simulink library "ann"  (Simulink 3.00)
undefined symbols (not defined in the file): V0, W0
libraries: simulink3 x3, neural x1
(part 1 of 2)
settings Model: LastModifiedBy=campa

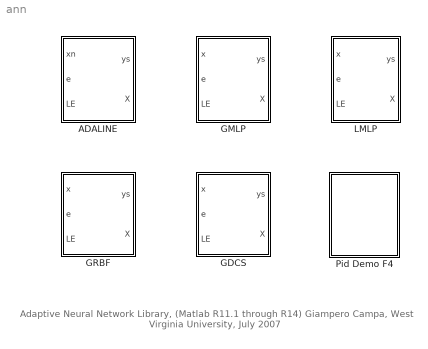
== system ann ==
  note: Adaptive Neural Network Library, (Matlab R11.1 through R14)
      | Giampero Campa, West Virginia University, July 2007
  ADALINE : Subsystem  mask(Adaline NN){dim=[4 1], eta=0.1, gam=1e-6, L=Inf, W=0, T=0.05}
      mask prompts: dim "[ni no]"; eta "Learning Rate"; gam "Stabilizing Factor"; L "Weight Limiter"; W "Initial Condition"; T "Sample Time"
      mask help: Self Adaptive Discrete Time MIMO Linear Neural Network
      mask init:
      | ni=dim(1);no=dim(2);
      mask Help:
      | <p>
      |   This Neural Network is used to adaptively approximate
      |   an affine vector field y=W*x+k, with the input vector
      |   x being a function of time.
      | </p>
      | <p>
      |   The first input is x. <br>
      |   The second input is the error signal (i.e. e=y-ys). <br>
      |   The third input is the learning enable:
      |        with LE=1 the learning is enabled,
      |        with LE=0 the learning is disabled.
      | </p>
      | <p>
      |   The first output is the learned function ys(x). <br>
      |   The second output is the states matrix reshaped columnwise. <br>
      | </p>
      | <p>
      |   The first parameter in the mask is a vector containing Ni and No,
      |   namely the dimensions (number of elements) of x and y.
      | </p>
      | <p>
      |   The second parameter in the mask is the learning rate.
      | </p>
      | <p>
      |   The third parameter in the mask is the stabilizing factor.
      | </p>
      | <p>
      |   The fourth parameter in the mask is a limiter for each element of the weight matrix.
      | </p>
      | <p>
      |   The initial condition could be either a vector of No*(Ni+1)
      |   parameters or a scalar. In the latter case, the scalar
      |   is repeated No*(Ni+1) times to form the initial condition vector.
      | </p>
      | <p>
      |   OUTPUT EQUATION: <br>
      |   At any given time t, if x(t) is the input vector,
      |   then the h-th output of the neural network is : <br>
      |   ys(h,t)=0.1*Wo(h,t)+Ws(h,t)*x(t) <br>
      |   where Wo(h,t) and Ws(h,t) are respectively the first element
      |   and the rest of the h-th row of the state matrix W(t). <br>
      | <br>
      |   STATE EQUATION (Learning Algorithm): <br>
      |   The state matrix W(t) is updated according to the gradient rule:
      |   W(t+T)=W(t)+eta*(dys/dW)*e(t)-eta*gamma*W(t) <br>
      |   where eta is the learning rate, dys/dW is a jacobian matrix,
      |   gamma is the stabilizing factor (sigma modification),
      |   e(t)=y(t)-ys(t) is the error vector at time t, and T is the sampling time.
      | </p>
      | <p>
      |   The final mask parameter is the sampling time of the block, T.
      | </p>
      | <p>
      |   This block is implemented in Simulink,
      |   to use it you should have the smxl library in your path.
      |   For further reference see some papers on the ADALINE NN.<br>
      | </p>
      | <p>
      |   Giampiero Campa, June 20 2003
      | </p>
  GDCS : Subsystem  mask(GDCS NN){Dim=[4 1], norlat=[50     0.2        0.01    600       0.99    0.005], eta=[0.03  0.003  0.1  0.001   0 ], lim=[1 1 1]*1e6, lga=on, S=zeros(1*(50*(50+4+5)+2),1), T=0.05}
      mask prompts: Dim "[Ni No]"; norlat "[Nmax Overlap RsThr Lambda Alpha Theta]"; eta "[Epsb Epsn etaW etaS etaC]"; lim "[limW limS limC]"; lga "Piecewise Conical Activation Function (otherwise Gaussian)"; S "Initial Condition, size = (Nmax*(Nmax+Ni+5)+2)*No"; T "Sample Time"
      mask help: Self Adaptive Discrete Time Generalized DCS Neural Network
      mask init:
      | if prod(size(Dim))==1,Dim=[Dim 1]; end
      mask Help:
      | <p>
      |   This Neural Network is used to adaptively approximate
      |   a vector field y=f(x), where x(t) is a vector of size Ni,
      |   and y(t) is a vector of size No.
      | </p>
      | <p>
      |   The first input is x (normally but not necessarily
      |   scaled between -1 and 1).<br>
      |   The second input is the error signal (i.e. e=y-ys).<br>
      |   The third input is the learning enable:
      |        with LE=1 the learning is enabled,
      |        with LE=0 the learning is disabled.
      | </p>
      | <p>
      |   The first output is the learned function ys(x). <br>
      |   The second output is the states matrix reshaped columnwise.
      |   Note that the network has in total No*(Nmax*(Nmax+Ni+5)+2) states,
      |   where Nmax is the maximum number of neurons per output.
      | </p>
      | <p>
      |   The first parameter in the mask is a vector containing Ni and No,
      |   namely the dimensions (number of elements) of x and y.
      | </p>
      | <p>
      |   The second parameter is a vector containing:<br>
      |   1) Nmax : the maximum number of active neurons for a single output.
      |       The total maximum number of active neurons in the whole network
      |       is this value multplied by the number of outputs, that is Nmax*No. <br>
      |   2) Overlapping Factor (when a new neuron is activated, the sigma (width) of
      |       this new neuron, is the sum of the distances from the two nearest
      |       neurons multiplied by the overlapping factor). <br>
      |   3) Resource Threshold, a new neuron is added only if the
      |       resource is greater than than this threshold. <br>
      |   4) Lambda, is the number of steps between insertion,
      |       a new neuron is activated only if the number of steps
      |       from the last activation is greater than lambda. <br>
      |   5) Alpha, is the connection weight decay constant
      |       for the neighborhood of the best matching unit.<br>
      |   6) Theta is the connection deletion threshold, that is when
      |       the weight falls below this threshold, it is set to 0,
      |       so the neuron is deactivated.
      | </p>
      | <p>
      |   The third parameters is 5 elements vector containing : <br>
      |   1) The two Kohonen update coefficients for the best
      |   matching unit and its neighborhood <br>
      |   2) the three learning rates for all the neurons states:
      |   weights, sigmas, and centers.
      | </p>
      | <p>
      |   The fifth parameter contains 3 limits for each element of the weight,
      |    sigma and center matrices. Basically, a limiting mechanism is implemented
      |    within the code so that the norms of each element of the weight, sigma
      |    and center vectors are confined within the upper bound entered as    parameter.
      | </p>
      | <p>
      |   The fifth parameter decides wether the activation function is
      |    piecewise conical or gaussian
      | </p>
      | <p>
      |   The initial condition must be a vector of size
      |   No*(Nmax*(Nmax+Ni+5)+2). If its norm is zero, then an
      |   appropriate initial condition (two neurons near zero) is chosen.
      | </p>
      | <p>
      |   STATE VECTOR MEANING: <br>
      |   Each output h is related to a contiguous vector of Nmax*(Nmax+Ni+5)+2
      |   states that are organized as follows: <br>
      |   ofY + 1 counter :  counts sampling times since last neuron activation. <br>
      |   ofY + 1 + [1..Nmax*Nmax] : interlayer connection matrix. <br>
      |   ofY + 1 + Nmax*Nmax + [1..Nmax*Ni] : neurons centers <br>
      |   ofY + 1 + Nmax*(Nmax+Ni) + [1..Nmax]: neurons weigths <br>
      |   ofY + 1 + Nmax*(Nmax+Ni+1) + [1..Nmax] : neurons sigmas (widths) <br>
      |   ofY + 1 + Nmax*(Nmax+Ni+2) + [1..Nmax] : neurons cumulative resource <br>
      |   ofY + 1 + Nmax*(Nmax+Ni+3) + [1..Nmax] : neurons resource<br>
      |   ofY + 1 + Nmax*(Nmax+Ni+4) + [1..Nmax] : number of times that each neuron has been bmu <br>
      |   ofY + 1 + Nmax*(Nmax+Ni+5) + 1 : number of active neurons <br>
      |   where ofY=(h-1)*(Nmax*(Nmax+Ni+5)+2) is the offset related to the h-th output.<br>
      |   It is important to note that the states related to a certain output
      |   are independent from the states related to a different output.
      |   Also note that the states related to the sigmas are only used for gaussian activation functions.
      | </p>
      | <p>
      |   BRIEF EXPLANATION OF THE ALGORITHM: <br>
      |   This Neural Network is essentially an RBF Neural Network with an
      |   additional lateral connection structure between the neural units
      |   of the hidden layer. This structure is used in an attempt to mirror
      |   the topology of the input manifold. <br>
      |   As in the RAN, the learning algorithm, in order to decrease the error,
      |   changes weights, positions and widths of the basis functions.
      |   The estimation error e(k) is accumulated locally to each neuron and
      |   used to determine where (and if) to activate a new neuron. <br>
      |   DSC stands for Dynamic Cell Structure.<br>
      | <br>
      |   OUTPUT EQUATION: <br>
      | At any given time t, if x(t) is the input vector, we indicate with bmu the nearest unit (among those related to the h-th output) to the current position of the input, and with sec is the nearest unit after the bmu. The neighborhood of the bmu is defined as the set of all the units that are connected to the bmu
      | by the interlayer connection matrix CN, that is all the units i such that CN(h,t,bmu,i) > 0.
      | Being W(h,t,bmu) and W(h,t,sec) the weights associated with the bmu and the sec units, and dist(bmu,x)  and dist(sec,x) their distances from the current input point x(t), if the PIECEWISE CONICAL activation functions are used, then the h-th output of the neural network is :
      | ys(h,t)=W(h,t,bmu) if dist(sec,x)>dist(sec,bmu)
      | ys(h,t)=W(h,t,bmu)+b*(W(h,t,sec)-W(h,t,bmu)) otherwise
      | where b=dist(bmu,x)/(dist(bmu,x)+dist(sec,x))
      | <br>
      |   If the GAUSSIAN activation functions are used t, then the h-th output
      |   of the neural network is simply: <br>
      |   ys(h,t)=W(h,t)*g(x(t),S(h,t),C(h,t)) <br>
      |   where W(h,t) is the output weight matrix related to the h-th output,
      |   g is the vector of radial basis functions of the input x(t), and
      |   finally S(h,t) and C(h,t) are vectors of widths and centers
      |   (relative to the h-th output).<br>
      | <br>
      |   STATE EQUATION (Learning Algorithm): <br>
      |   Being e(h,t)=y(h,t)-ys(h,t) the h-th element of the error vector,
      |   at a time t, and x(t) the input vector at the same time, we indicate
      |   with bmu the nearest unit (among those related to the h-th output)
      |   to the current position of the input, and with sec is the nearest
      |   unit after the bmu. The neighborhood of the bmu is defined as the set of
      |   all the units that are connected to the bmu by the interlayer connection
      |   matrix CN, that is all the units i such that CN(h,t,bmu,i) > 0. <br>
      |   Firstly, the connection matrix updated, by setting to 1 the strength of
      |   the connection between bmu and sec, ( that is CN(h,t+1,bmu,sec)=1 and
      |   CN(h,t+1,sec,bmu)=1 ), and by multiplying by a value alpha < 1 the
      |   strength of all the other connections ( that is for every i,j <> bmu,sec
      |   CN(h,t+1,i,j)=CN(h,t,i,j)*alpha ). Also, all the connections whose
      |   strength is less than a threshold theta are deleted (i.e. their strength
      |   is set to 0). This kind of updating is also called "Hebbian Learning". <br>
      |   The next step in the network adaptation algorithm consist in moving the
      |   positions of the BMU and its neighborhood toward the current input x(t),
      |   following a so called "Kohonen" rule. Specifically, if C(h,t,i) is
      |   the position of the neuron i, related to the output h, at time t,
      |   then for each neuron i belonging to the neighborhood of the bmu
      |   we have C(h,t+1,i)=epsilon(i)*(x(t)-C(h,t,i)). <br>
      |   Each neuron i is associated with a value called resource, R(h,t,i) and
      |   at this point in the algorithm, the resource of the bmu is updated,
      |   specifically, the resource of the bmu is set to the error e(h,t)
      |   divided by the number of times that the unit has been selected as bmu. <br>
      |   If the mean value of the resource of the whole network is greater than
      |   a certain threshold RsThr, and if the last neuron activation was more than
      |   lambda steps ago, then a new neuron is activated. <br>
      |   The new neuron n is placed between the position of the unit with highest
      |   resource w and the position of the unit with highest resource within the
      |   neighborhood of w, excluding w itself, let us indicate it with v.
      |   In detail, C(h,t+1,n)=C(h,t,w)+b*(C(h,t,v)-C(h,t,w)), where
      |   b=R(h,t,w)/(R(h,t,w)+R(h,t,v)). <br>
      |   The interlayer connections from w to n and from n to v are set to 1,
      |   the original connection between w and v is set to 0. Both resource and
      |   weight of the new neuron are computed by interpolating the resource and
      |   weight of the two neurons w and v:  <br>
      |   R(h,t+1,n)=R(h,t,w)+b*(R(h,t,v)-R(h,t,w)) <br>
      |   W(h,t+1,n)=W(h,t,w)+b*(W(h,t,v)-W(h,t,w)) <br>
      |   The width of the basis function of n is set to
      |   S(h,t,n)=overlap*(C(h,t,v)-C(h,t,w)), where overlap is the so called
      |   overlapping factor. <br>
      |   Finally, as a last step of the adaptation algorithm, the vector X(t)
      |   containing all the neural network weights and widths,
      |   is updated according to the gradient rule: <br>
      |   X(t+T)=X(t)+eta*(dys/dX)*e(t) <br>
      |   where eta is the learning rate, dys/dX is a jacobian matrix,
      |   and T is the sampling time.
      | </p>
      | <p>
      |   The final mask parameter is the sampling time of the block, T.
      | </p>
      | <p>
      |   This block calls the mex file obtained by compiling the s-function
      |   dcsgl.c, therefore, to use the block, you should have the resulting
      |   mex file (on windows platform the file is dcsgl.dll) in the matlab path.<br>
      |   For further reference see some papers on DSC Networks.<br>
      | </p>
      | <p>
      |   Giampiero Campa, January 2007
      | </p>
  GMLP : Subsystem  mask(GMLP NN){dim=[4 10 1], eta=[0.003 0.003 0.003]/10, L=[inf inf inf], alp=0.01, ini=1, T=0.05}
      mask prompts: dim "[ni nh no]"; eta "[etaV etaW etaP]"; L "[Lv Lw Lp] (Weight Limiters)"; alp "Momentum (alpha)"; ini "Initial Conditions"; T "Sample Time"
      mask help: Self Adaptive Discrete Time Generalized MLP Neural Network
      mask init:
      | ni=dim(1);nh=dim(2);no=dim(3);
      | ns=nh*ni+no*nh+4*no+4*nh;
      | etaV=eta(1);
      | etaW=eta(2);
      | etaP=eta(3);
      | 
      | if size(ini)==[1 1],
      |    V0 = ini*reshape( rand(nh,ni)-0.5 ,nh*ni,1 );
      |    W0 = ini*reshape( rand(no,nh)-0.5 ,no*nh,1 );
      |    Gm0 = ini*(rand(no,1) - 0.5);
      |    Uo0=   ones(no,1);
      |    Lo0=-1*ones(no,1);
      |    To0=   ones(no,1);
      |    Te0 = ini*(rand(nh,1) - 0.5);
      |    Uh0=   ones(nh,1);
      |    Lh0=-1*ones(nh,1);
      |    Th0=   ones(nh,1);
      | 
      |   x0=[V0;W0;Gm0;Uo0;Lo0;To0;Te0;Uh0;Lh0;Th0];
      |   d0=x0*0;
      | 
      | elseif size(ini)==[2*ns 1],
      |   x0=ini(1:ns);
      |   d0=ini(ns+1:2*ns);
      | else
      |    warning(['The initial condition size must be 1 by 1 or ' mat2str(2*ns) ' by 1']);
      | end
      mask Help:
      | <p>
      |   This Neural Network is used to adaptively approximate
      |    a (possibly nonlinear) vector field y=f(x),
      |    with the input vector x being a function of time.
      | </p>
      | <p>
      |   The first input is x. <br>
      |   The second input is the error signal (i.e. e=y-ys). <br>
      |   The third input is the learning enable: <br>
      |        with LE=1 the learning is enabled,
      |        with LE=0 the learning is disabled.
      | </p>
      | <p>
      |   The first output is the learned function ys(x).<br>
      |   The second output is the states matrix reshaped columnwise.
      | </p>
      | <p>
      |   The first parameter in the mask is a vector containing respectively
      |   the number of inputs Ni, the number of neurons in the hidden layer Nh,
      |   and the number of outputs No.<br>
      |   The second parameter contains the learning rates for:<br>
      |    1) the weights connecting input and hidden layers (V)<br>
      |    2) the weights connecting hidden and output layers (W)<br>
      |    3) the vector of parameters [Pw Uo Lo To Pv Uh Lh Th]<br>
      |   The next parameter contains limiters for each element of the 3 items
      |    in the above list. Basically, a limiting mechanism is implemented
      |    within the code so that  each element of V,W and the vector
      |    [Pw Uo Lo To Pv Uh Lh Th] is always limited.<br>
      |    Finally, the fourth parameter is the so called momentum.
      | </p>
      | <p>
      |   The initial condition could be a vector of size
      |   2*(Nh*(Ni+No)+4*(No+Nh)), or a scalar, in the latter
      |   case, the scalar multiplies the weights of an
      |   appropriate random initial condition vector.
      | </p>
      | <p>
      |   STATE VECTOR MEANING: <br>
      |   The state is a column vector composed by 2 contiguous
      |   parts having both Nh*(Ni+No)+4*(No+Nh) elements. <br>
      |   The states in the first part are organized as follows: <br>
      |   [1..Nh*Ni] : weights connecting the input to the hidden layer. <br>
      |   Nh*Ni+[1..No*Nh] : weights connecting the hidden layer to the output layer. <br>
      |   Nh*Ni+No*Nh+[1..No] : hidden layer to output threshold vector (Pv).<br>
      |   Nh*Ni+No*Nh+No+[1..No] : upper limits of the output layer base functions (Uo).<br>
      |   Nh*Ni+No*Nh+2*No+[1..No] : lower limits of the output layer base functions (Lo).<br>
      |   Nh*Ni+No*Nh+3*No+[1..No] : slopes of the output layer base functions (To).<br>
      |   Nh*Ni+No*Nh+4*No+[1..Nh] : input to hidden layer threshold vector (Pw).<br>
      |   Nh*Ni+No*Nh+4*No+Nh+[1..Nh] : upper limits of the hidden layer base functions (Uh).<br>
      |   Nh*Ni+No*Nh+4*No+2*Nh+[1..Nh] : lower limits of the hidden layer base functions (Lh).<br>
      |   Nh*Ni+No*Nh+4*No+3*Nh+[1..Nh] : slopes of the hidden layer base functions (Th).<br>
      |   The second half of the state vector contains the states of an error filter
      |   that somehow represents the past increments of the first half of the state vector.
      |   See below in the "state equation" section for a more detailed explanation of this.
      | </p>
      | <p>
      |   BRIEF EXPLANATION OF THE ALGORITHM: <br>
      |   This Neural Network is essentially a 2-layered sigmoidal Neural Network,
      |   in which the usual sigmoidal base function is replaced by a more flexible
      |   function:  <br> f(s) = L + (U-L)/(1+exp(-s/T)) <br>
      |   where s is the (scalar) input to the function,
      |   L is the lower limit, U the upper limit, and T the slope.<br>
      |   The function reduces to the usual sigmoid when L=0, U=1 and T=1.<br>
      |   Two affine transformations (i.e. having the form y=A*x+b) connect
      |   the input to the hidden layer and the hidden layer to the output layer. <br>
      |   The learning algorithm allows the parameters A,b,L,U,T for each layer to
      |   change. An extended gradient rule, structured according to the well known
      |   backpropagation algorithm, is used to update the parameters. <br>
      |   The acronym GMLP stands for Generalized Multi Layer Perceptron,
      |   and it is used to refer to this kind of neural network architectures.
      | <br>
      | <br>
      |   OUTPUT EQUATION: <br>
      |   At any given time t, if x(t) is the input vector, then the i-th
      |   element of the output vector AT THE HIDDEN LAYER is:
      |   z(i,t) = Lh(i,t) + (Uh(i,t)-Lh(i,t))/(1+exp(-( V(i,t)*x(t)+Pv(i,t) )/Th(i,t)))
      |   where Lh(i,t) is the i-th element of the lower limit vector (for the hidden layer),
      |   Uh(i,t) is the i-th element of the upper limit vector (for the hidden layer),
      |   Th(i,t) is the i-th element of the slope vector (for the hidden layer),
      |   V(i,t) is the i-th row of the (input to hidden layer) weight matrix,
      |   and Pv(i,t) is the i-th element of the (input to hidden layer) threshold vector. <br>
      |   The i-th element of the output vector AT THE NETWORK OUTPUT is:
      |   ys(i,t) = Lo(i,t) + (Uo(i,t)-Lo(i,t))/(1+exp(-( W(i,t)*z(t)+Pw(i,t) )/To(i,t)))
      |   where Lo(i,t) is the i-th element of the lower limit vector (for the output layer),
      |   Uo(i,t) is the i-th element of the upper limit vector (for the output layer),
      |   To(i,t) is the i-th element of the slope vector (for the output layer),
      |   W(i,t) is the i-th row of the (hidden layer to output) weight matrix,
      |   and Pw(i,t) is the i-th element of the (hidden layer to output) threshold vector.
      | <br><br>
      |   STATE EQUATION (Learning Algorithm): <br>
      |   Being e(t)=y(t)-ys(t) the error vector at time t, the vector X(t)
      |   containing the first Nh*(Ni+No)+4*(No+Nh) neural network states
      |   is updated according to an "extended" gradient rule: <br>
      |   X(t+T)=X(t)+eta*(dys/dX)*e(t)+Z(t) <br>
      |   where eta is the learning rate, dys/dX is the jacobian matrix,
      |   T is the sampling time, and Z(t) represents an additional
      |   contribution from a filtered error:<br>
      |   D(t+1)=alpha*D(t)-eta*(dys/dX)*e(t) <br>
      |   Z(t)=alpha*D(t) <br>
      |   The filter decay rate, alpha, is called "momentum", if alpha=0,
      |   the update law reduces to the classic gradient rule.<br>
      |   It can be seen Z(t) somehow represents all the past increments of X(t).<br>
      |   The final part of the whole state vector is D(t).
      | </p>
      | <p>
      |   The final mask parameter is the sampling time of the block, T.
      | </p>
      | <p>
      |   This block is implemented in Simulink,
      |   to use it you should have the smxl library in your path.
      |   For further reference see some papers on the backpropagation
      |   algorithm applied to multilayer sigmoidal neural networks.<br>
      | </p>
      | <p>
      |   Giampiero Campa, 2007
      | </p>
  GRBF : Subsystem  mask(GRBF NN){dim=[4 1], nwrap=[100     1           10               1], eta=[1 1 1]*1e-3, gam=[1 1 1]*1e-6, lim=[1 1 1]*1e6, e1=0.2, e2=[0.3  0.2  0.999], e3=[0 0.5], x0=zeros((4+2)*100+2,1), T=0.05}
      mask prompts: dim "Dimensions [Ni No]"; nwrap "[Nmax Overlap Radius Prune]"; eta "Learning Rates [weight,sigma,center]"; gam "Stabilizing Factors [weight,sigma,center]"; lim "Limiters [weight,sigma,center]"; e1 "Threshold For Error (Criteria #1)"; e2 "Center Distance [Emax Emin Egam] (Criteria #2)"; e3 "Threshold and Pole for Filtered Error (Criteria #3)"; x0 "Initial Condition, size = ((Ni+2)*Nmax+2)*No"; T "Sample Time"
      mask help: Self Adaptive Discrete Time Generalized RBF Neural Network
      mask Help:
      | <p>
      |   This Neural Network is used to adaptively approximate
      |   a vector field y=f(x), where x(t) is a vector of size Ni,
      |   and y(t) is a vector of size No.
      | </p>
      | <p>
      |   The first input is x (normally but not necessarily
      |   scaled between -1 and 1).<br>
      |   The second input is the error signal (i.e. e=y-ys).<br>
      |   The third input is the learning enable:
      |        with LE=1 the learning is enabled,
      |        with LE=0 the learning is disabled.
      | </p>
      | <p>
      |   The first output is the learned function ys(x). <br>
      |   The second output is the states matrix reshaped columnwise.
      |   Note that the network has in total ((Ni+2)*Nmax+2)*No states,
      |   where Nmax is the maximum number of neurons per output.
      | </p>
      | <p>
      |   The first parameter in the mask is a vector containing Ni and No,
      |   namely the dimensions (number of elements) of x and y.
      | </p>
      | <p>
      |   The second parameter is a vector containing:<br>
      |   1) Nmax : the maximum number of active neurons for a single output.
      |       The total maximum number of active neurons in the whole network
      |       is this value multplied by the number of outputs, that is Nmax*No<br>
      |   2) Overlapping Factor (when a new neuron is activated, the sigma (width) of
      |       this new neuron, is the distance from the nearest neuron multiplied by the
      |       overlapping factor).<br>
      |   3) Radius, is the radius of the ipersphere inside which the neurons
      |       are updated. Note that the radius only influences the updating
      |       (learning) but does not concern the output computation.<br>
      |   5) Pruning, when 1, it enables the network to prune the
      |       worst neuron to allocate a new one after the
      |       maximum number of neurons has been reached. <br>
      | </p>
      | <p>
      |   The third parameter contains the 3 learning rates for
      |   all the neuron states: weights, sigmas, and centers.
      | </p>
      | <p>
      |   The fourth parameter contains the 3 stabilizing factors
      |   (Sigma Modifications) for weights, sigmas, and centers.
      |   When the learning is enabled (LE=1), these parameters
      |   counteract casual drifting by slowly driving weights, sigmas,
      |   and centers towards zero with a negative feedback gain
      |   equal to the learning rate by the stabilizing factor.
      |   Look further on, in the algorithm explanation section,
      |   to get an idea on how this works.
      | </p>
      | <p>
      |   The fifth parameter contains 3 limits for each element of the weight,
      |    sigma and center matrices. Basically, a limiting mechanism is implemented
      |    within the code so that the norms of each element of the weight, sigma
      |    and center vectors are confined within the upper bound entered as parameter.
      | </p>
      | <p>
      |   The sixth parameter is the threshold for the error, a new neuron
      |   (related to the h-th output) is added in the current x(t) position
      |   only if the h-th element of the error is greater than this threshold).
      | </p>
      | <p>
      |   The seventh parameter is a vector containing the maximum and
      |   minimum thresholds for the distance, as well as the decay factor.
      |   At any given instant t, the actual threshold is
      |   max(Emax*Egam^t,Emin), that is, the threshold starts from Emax
      |   and goes to Emin with an exponential decay Egam. <br>
      |   A new neuron (to approximate the h-th output) is added in
      |   the current x(t) position only if the distance from the nearest
      |   (h-th output related) neuron is greater than this threshold. <br>
      | </p>
      | <p>
      |   The eight parameter is a vector containing the threshold
      |   for the filtered error, and the pole of the linear filter: <br>
      |   ef(h,t+1)=Pole*ef(h,t)+(1-Pole)*(y(h,t)-ys(h,t)) <br>
      |   A new neuron, related to the h-th output, is added in the
      |   current position x(t) only if the h-th element of the
      |   filtered error ef(h,t) is greater than this threshold.
      | </p>
      | <p>
      |   The initial condition must be a vector of size
      |   ((Ni+2)*Nmax+2)*No. If its norm is zero, then an
      |   appropriate initial condition (one single neuron at zero) is chosen.
      | </p>
      | <p>
      |   STATE VECTOR MEANING: <br>
      |   Each output h is related to a contiguous vector of (Ni+2)*Nmax+2
      |   states that are organized as follows: <br>
      |   ofY + [1..Nmax*Ni] : neurons positions <br>
      |   ofY + [Nmax*Ni+1..Nmax*(Ni+1)] : neurons sigma <br>
      |   ofY + [Nmax*(Ni+1)+1..Nmax*(Ni+2)] : neurons weigths <br>
      |   ofY +  Nmax*(Ni+2)+1 : number of active neurons <br>
      |   ofY +  Nmax*(Nu+2)+2 : current value of the filtered error ef(k) <br>
      |   where ofY=(h-1)*((Ni+2)*Nmax+2) is the offset related to the h-th output.<br>
      |   It is important to note that the states related to a certain output
      |   are independent from the states related to a different output.
      | </p>
      | <p>
      |   BRIEF EXPLANATION OF THE LEARNING ALGORITHM: <br>
      |   This Neural Network is a Generalized RBF Neural Network in which
      |   the learning algorithm, in order to decrease the error, not only
      |   changes weights, positions and widths of the basis functions,
      |   but it also adds neurons when and where they are needed most.<br>
      |   Tha algorithm is also called EMRAN, which stands for
      |    "Extended Minimal Resource Allocating Network".<br>
      | <br>
      |   OUTPUT EQUATION: <br>
      |   At any given time t, if x(t) is the input vector,
      |   then the h-th output of the neural network is : <br>
      |   ys(h,t)=W(h,t)*g(x(t),S(h,t),C(h,t)) <br>
      |   where W(h,t) is the output weight matrix related to the h-th output,
      |   g is the vector of radial basis functions of the input x(t), and
      |   finally S(h,t) and C(h,t) are vectors of widths and centers
      |   (relative to the h-th output).<br>
      | <br>
      |   STATE EQUATION (Learning Algorithm): <br>
      |   Being e(h,t)=y(h,t)-ys(h,t) the h-th element of the error vector,
      |   at a time t, a neuron is added if and only if ALL the following criteria are met: <br>
      |   1) the error e(h,t) is greater than a threshold (E1). <br>
      |   2) the distance from the nearest neuron is greater than a threshold (E2). <br>
      |   3) the filtered error ef(h,t) is greater than a threshold. <br>
      |   This new neuron j is positioned at the current input point C(h,t+1,j)=x(t),
      |   the width of its basis function is set to S(h,t+1,j)=overlap*dist(x(t),C(h,t,nearest)),
      |   that is, an overlapping factor multiplied by the distance to the nearest neuron.
      |   Finally, its output weight vector Wj(h,t) is initialized to e(h,t).<br>
      |   If at least one of the three criteria is not satisfied, then the vector X(t)
      |   containing all the neural network states, (weights, widths, and centers)
      |   is updated according to the modified gradient rule: <br>
      |   X(t+T)=X(t)+eta*(dys/dX)*e(t)-eta*gamma*X(t) <br>
      |   where eta is the learning rate, dys/dX is a jacobian matrix,
      |   gamma is the stabilizing factor (sigma modification),
      |   and T is the sampling time.
      | </p>
      | <p>
      |   The final mask parameter is the sampling time of the block, T.
      | </p>
      | <p>
      |   This block calls the mex file obtained by compiling the s-function
      |   emran6.c, therefore, to use the block, you should have the resulting
      |   mex file (on windows platform the file is emran.dll) in the matlab path.<br>
      |   For further reference see some papers on EMRAN-RBF.<br>
      | </p>
      | <p>
      |   Giampiero Campa, June 4 2003
      | </p>
  LMLP : Subsystem  mask(Adaptive Neural Network){s=[4  10  1], g=[0.4 0.4 0.01 1 1], lim=[1e37 1e37], k=[0.01  0.1  0.1], w0=0.01, v0=0.01, T=0.05}
      mask prompts: s "[ni nh no] (Number of inputs, hidden layer neurons, and outputs)"; g "[G F lambda act bias] (Learning rates, activation, and bias)"; lim "[limW limV] (Weight Limiters)"; k "[Kv  Z_bar  Kz] (Robustifying terms)"; w0 "Initial Conditions: W(0) (scalar = magnitude of a random matrix)"; v0 "Initial Conditions: V(0) (scalar = magnitude of a random matrix)"; T "Sample Time"
      mask help: Lewis Multi Layer Perceptron
      mask init:
      | nni=s(1);nnh=s(2);nno=s(3); G=g(1);F=g(2);lam=g(3);a=g(4);bias=g(5);
      | Kv=k(1); Z_bar=k(2);Kz=k(3);LW=lim(1);LV=lim(2);
      | if size(w0,1)*size(w0,2)==1 & nnh*nno>1, W0=w0*rand(nnh*nno,1);end
      | if size(v0,1)*size(v0,2)==1 & nni*nnh >1, V0=v0*rand(nni*nnh,1);end
      mask Help:
      | <html xmlns:o="urn:schemas-microsoft-com:office:office"
      | xmlns:w="urn:schemas-microsoft-com:office:word"
      | xmlns="http://www.w3.org/TR/REC-html40">
      | 
      | <head>
      | <meta http-equiv=Content-Type content="text/html; charset=windows-1252">
      | <meta name=ProgId content=Word.Document>
      | <meta name=Generator content="Microsoft Word 9">
      | <meta name=Originator content="Microsoft Word 9">
      | <link rel=File-List href="./LMLP3_files/filelist.xml">
      | <title>Notation and adaptation algorithm are taken from the paper:</title>
      | <!--[if gte mso 9]><xml>
      |  <o:DocumentProperties>
      |   <o:Author>Control Lab</o:Author>
      |   <o:LastAuthor>Richard Feynman</o:LastAuthor>
      |   <o:Revision>8</o:Revision>
      |   <o:TotalTime>170</o:TotalTime>
      |   <o:Created>2007-01-22T15:43:00Z</o:Created>
      |   <o:LastSaved>2007-01-22T16:20:00Z</o:LastSaved>
      |   <o:Pages>1</o:Pages>
      |   <o:Words>293</o:Words>
      |   <o:Characters>1671</o:Characters>
      |   <o:Company>GA TECH</o:Company>
      |   <o:Lines>13</o:Lines>
      |   <o:Paragraphs>3</o:Paragraphs>
      |   <o:CharactersWithSpaces>2052</o:CharactersWithSpaces>
      |   <o:Version>9.2720</o:Version>
      |  </o:DocumentProperties>
      | </xml><![endif]--><!--[if gte mso 9]><xml>
      |  <w:WordDocument>
      |   <w:Zoom>75</w:Zoom>
      |  </w:WordDocument>
      | </xml><![endif]-->
      | <style>
      | <!--
      |  /* Style Definitions */
      | p.MsoNormal, li.MsoNormal, div.MsoNormal
      | 	{mso-style-parent:"";
      | 	margin:0in;
      | 	margin-bottom:.0001pt;
      | 	mso-pagination:widow-orphan;
      | 	font-size:12.0pt;
      | 	font-family:"Times New Roman";
      | 	mso-fareast-font-family:"Times New Roman";}
      | p.MsoBodyText, li.MsoBodyText, div.MsoBodyText
      | 	{margin-top:0in;
      | 	margin-right:3.35in;
      | 	margin-bottom:0in;
      | 	margin-left:0in;
      | 	margin-bottom:.0001pt;
      | 	mso-pagination:widow-orphan;
      | 	font-size:12.0pt;
      | 	font-family:"Times New Roman";
      | 	mso-fareast-font-family:"Times New Roman";}
      | p.MsoBodyText2, li.MsoBodyText2, div.MsoBodyText2
      | 	{margin-top:0in;
      | 	margin-right:2.35in;
      | 	margin-bottom:0in;
      | 	margin-left:0in;
      | 	margin-bottom:.0001pt;
      | 	mso-pagination:widow-orphan;
      | 	font-size:12.0pt;
      | 	font-family:"Times New Roman";
      | 	mso-fareast-font-family:"Times New Roman";}
      | @page Section1
      | 	{size:8.5in 11.0in;
      | 	margin:1.0in 1.25in 1.0in 1.25in;
      | 	mso-header-margin:.5in;
      | 	mso-footer-margin:.5in;
      | 	mso-paper-source:0;}
      | div.Section1
      | 	{page:Section1;}
      |  /* List Definitions */
      | @list l0
      | 	{mso-list-id:387336931;
      | 	mso-list-type:hybrid;
      | 	mso-list-template-ids:1661509918 67698705 67698713 67698715 67698703 67698713 67698715 67698703 67698713 67698715;}
      | @list l0:level1
      | 	{mso-level-text:"%1\)";
      | 	mso-level-tab-stop:.5in;
      | 	mso-level-number-position:left;
      | 	text-indent:-.25in;}
      | @list l1
      | 	{mso-list-id:1390807613;
      | 	mso-list-type:hybrid;
      | 	mso-list-template-ids:210782786 67698705 67698713 67698715 67698703 67698713 67698715 67698703 67698713 67698715;}
      | @list l1:level1
      | 	{mso-level-text:"%1\)";
      | 	mso-level-tab-stop:.5in;
      | 	mso-level-number-position:left;
      | 	text-indent:-.25in;}
      | @list l2
      | 	{mso-list-id:1468430361;
      | 	mso-list-type:hybrid;
      | 	mso-list-template-ids:-783395272 67698705 67698713 67698715 67698703 67698713 67698715 67698703 67698713 67698715;}
      | @list l2:level1
      | 	{mso-level-text:"%1\)";
      | 	mso-level-tab-stop:.5in;
      | 	mso-level-number-position:left;
      | 	text-indent:-.25in;}
      | @list l3
      | 	{mso-list-id:2055232913;
      | 	mso-list-type:hybrid;
      | 	mso-list-template-ids:-1797358054 67698705 67698713 67698715 67698703 67698713 67698715 67698703 67698713 67698715;}
      | @list l3:level1
      | 	{mso-level-text:"%1\)";
      | 	mso-level-tab-stop:.5in;
      | 	mso-level-number-position:left;
      | 	text-indent:-.25in;}
      | @list l4
      | 	{mso-list-id:2063862014;
      | 	mso-list-type:hybrid;
      | 	mso-list-template-ids:756564476 67698705 67698713 67698715 67698703 67698713 67698715 67698703 67698713 67698715;}
      | @list l4:level1
      | 	{mso-level-text:"%1\)";
      | 	mso-level-tab-stop:.5in;
      | 	mso-level-number-position:left;
      | 	text-indent:-.25in;}
      | ol
      | 	{margin-bottom:0in;}
      | ul
      | 	{margin-bottom:0in;}
      | -->
      | </style>
      | </head>
      | 
      | <body lang=EN-US style='tab-interval:.5in'>
      | 
      | <div class=Section1>
      | 
      | <p class=MsoBodyText2 style='margin-right:-1.8pt'>The block implements a
      | Lewis-Type<span style="mso-spacerun: yes">  </span>MIMO Single Hidden Layer
      | Sigmoidal Neural Network.</p>
      | 
      | <p class=MsoNormal style='margin-right:-1.8pt'><![if !supportEmptyParas]>&nbsp;<![endif]><o:p></o:p></p>
      | 
      | <p class=MsoNormal style='margin-right:-1.8pt'>Notation and adaptation
      | algorithm are taken from the paper:</p>
      | 
      | <p class=MsoBodyText style='margin-right:-1.8pt'>F.L. Lewis, A. Yesildirek, and
      | K. Liu, Multilayer Neural-Net Robot Controller with Guaranteed Tracking Performance,
      | IEEE Transactions on Neural Networks 7 (1996), no. 2, 1-12.</p>
      | 
      | <p class=MsoBodyText style='margin-right:-1.8pt'><![if !supportEmptyParas]>&nbsp;<![endif]><o:p></o:p></p>
      | 
      | <p class=MsoBodyText style='margin-right:-1.8pt;tab-stops:27.0pt'>V<sub>dot<span
      | style='mso-tab-count:1'>   </span></sub>=<span style="mso-spacerun: yes">
      | </span>G[x<span style='font-family:Symbol;mso-ascii-font-family:"Times New Roman";
      | mso-hansi-font-family:"Times New Roman";mso-char-type:symbol;mso-symbol-font-family:
      | Symbol'><span style='mso-char-type:symbol;mso-symbol-font-family:Symbol'>z</span></span>W<sup>T</sup><span
      | style='font-family:Symbol;mso-ascii-font-family:"Times New Roman";mso-hansi-font-family:
      | "Times New Roman";mso-char-type:symbol;mso-symbol-font-family:Symbol'><span
      | style='mso-char-type:symbol;mso-symbol-font-family:Symbol'>s</span></span>’(V<sup>T</sup>x)
      | - <span style='font-family:Symbol;mso-ascii-font-family:"Times New Roman";
      | mso-hansi-font-family:"Times New Roman";mso-char-type:symbol;mso-symbol-font-family:
      | Symbol'><span style='mso-char-type:symbol;mso-symbol-font-family:Symbol'>l</span></span><span
      | style='font-family:Symbol;mso-ascii-font-family:"Times New Roman";mso-hansi-font-family:
      | "Times New Roman";mso-char-type:symbol;mso-symbol-font-family:Symbol'><span
      | style='mso-char-type:symbol;mso-symbol-font-family:Symbol'>ï</span></span><span
      | style='font-family:Symbol;mso-ascii-font-family:"Times New Roman";mso-hansi-font-family:
      | "Times New Roman";mso-char-type:symbol;mso-symbol-font-family:Symbol'><span
      | style='mso-char-type:symbol;mso-symbol-font-family:Symbol'>z</span></span><span
      | style='font-family:Symbol;mso-ascii-font-family:"Times New Roman";mso-hansi-font-family:
      | "Times New Roman";mso-char-type:symbol;mso-symbol-font-family:Symbol'><span
      | style='mso-char-type:symbol;mso-symbol-font-family:Symbol'>ï</span></span>V]</p>
      | 
      | <p class=MsoBodyText style='margin-right:-1.8pt;tab-stops:27.0pt'>W<sub>dot<span
      | style='mso-tab-count:1'>  </span></sub>=<span style="mso-spacerun: yes">
      | </span>F[(<span style='font-family:Symbol;mso-ascii-font-family:"Times New Roman";
      | mso-hansi-font-family:"Times New Roman";mso-char-type:symbol;mso-symbol-font-family:
      | Symbol'><span style='mso-char-type:symbol;mso-symbol-font-family:Symbol'>s</span></span>(V<sup>T</sup>x)-<span
      | style='font-family:Symbol;mso-ascii-font-family:"Times New Roman";mso-hansi-font-family:
      | "Times New Roman";mso-char-type:symbol;mso-symbol-font-family:Symbol'><span
      | style='mso-char-type:symbol;mso-symbol-font-family:Symbol'>s</span></span>’(V<sup>T</sup>x)V<sup>T</sup>x)<span
      | style='font-family:Symbol;mso-ascii-font-family:"Times New Roman";mso-hansi-font-family:
      | "Times New Roman";mso-char-type:symbol;mso-symbol-font-family:Symbol'><span
      | style='mso-char-type:symbol;mso-symbol-font-family:Symbol'>z</span></span> - <span
      | style='font-family:Symbol;mso-ascii-font-family:"Times New Roman";mso-hansi-font-family:
      | "Times New Roman";mso-char-type:symbol;mso-symbol-font-family:Symbol'><span
      | style='mso-char-type:symbol;mso-symbol-font-family:Symbol'>l</span></span><span
      | style='font-family:Symbol;mso-ascii-font-family:"Times New Roman";mso-hansi-font-family:
      | "Times New Roman";mso-char-type:symbol;mso-symbol-font-family:Symbol'><span
      | style='mso-char-type:symbol;mso-symbol-font-family:Symbol'>ï</span></span><span
      | style='font-family:Symbol;mso-ascii-font-family:"Times New Roman";mso-hansi-font-family:
      | "Times New Roman";mso-char-type:symbol;mso-symbol-font-family:Symbol'><span
      | style='mso-char-type:symbol;mso-symbol-font-family:Symbol'>z</span></span><span
      | style='font-family:Symbol;mso-ascii-font-family:"Times New Roman";mso-hansi-font-family:
      | "Times New Roman";mso-char-type:symbol;mso-symbol-font-family:Symbol'><span
      | style='mso-char-type:symbol;mso-symbol-font-family:Symbol'>ï</span></span>W]</p>
      | 
      | <p class=MsoBodyText style='margin-right:-1.8pt;tab-stops:27.0pt'>v<sub>ad<span
      | style='mso-tab-count:1'>    </span></sub>=<span style="mso-spacerun: yes">
      | </span>W<sup>T</sup><span style='font-family:Symbol;mso-ascii-font-family:"Times New Roman";
      | mso-hansi-font-family:"Times New Roman";mso-char-type:symbol;mso-symbol-font-family:
      | Symbol'><span style='mso-char-type:symbol;mso-symbol-font-family:Symbol'>s</span></span>(V<sup>T</sup>x)</p>
      | 
      | <p class=MsoBodyText style='margin-right:-1.8pt;tab-stops:27.0pt'>v<sub>bar<span
      | style='mso-tab-count:1'>   </span></sub>= -K<sub>v</sub> (<span
      | style='font-family:Symbol;mso-ascii-font-family:"Times New Roman";mso-hansi-font-family:
      | "Times New Roman";mso-char-type:symbol;mso-symbol-font-family:Symbol'><span
      | style='mso-char-type:symbol;mso-symbol-font-family:Symbol'>ï</span></span>Z<span
      | style='font-family:Symbol;mso-ascii-font-family:"Times New Roman";mso-hansi-font-family:
      | "Times New Roman";mso-char-type:symbol;mso-symbol-font-family:Symbol'><span
      | style='mso-char-type:symbol;mso-symbol-font-family:Symbol'>ï</span></span><sub>F</sub>
      | + Z<sub>bar</sub>)<span style='font-family:Symbol;mso-ascii-font-family:"Times New Roman";
      | mso-hansi-font-family:"Times New Roman";mso-char-type:symbol;mso-symbol-font-family:
      | Symbol'><span style='mso-char-type:symbol;mso-symbol-font-family:Symbol'>z</span></span><sup>T</sup>
      | - K<sub>z</sub><span style='font-family:Symbol;mso-ascii-font-family:"Times New Roman";
      | mso-hansi-font-family:"Times New Roman";mso-char-type:symbol;mso-symbol-font-family:
      | Symbol'><span style='mso-char-type:symbol;mso-symbol-font-family:Symbol'>z</span></span><sup>T</sup></p>
      | 
      | <p class=MsoBodyText style='margin-right:-1.8pt'><![if !supportEmptyParas]>&nbsp;<![endif]><o:p></o:p></p>
      | 
      | <p class=MsoNormal style='margin-right:-1.8pt'>The <u>Inputs</u> are:</p>
      | 
      | <p class=MsoNormal style='margin-top:0in;margin-right:-1.8pt;margin-bottom:
      | 0in;margin-left:.5in;margin-bottom:.0001pt;text-indent:-.25in;mso-list:l2 level1 lfo2;
      | tab-stops:list .5in'><![if !supportLists]>1)<span style='font:7.0pt "Times New Roman"'>&nbsp;&nbsp;&nbsp;
      | </span><![endif]>net input vector x.</p>
      | 
      | <p class=MsoNormal style='margin-top:0in;margin-right:-1.8pt;margin-bottom:
      | 0in;margin-left:.5in;margin-bottom:.0001pt;text-indent:-.25in;mso-list:l2 level1 lfo2;
      | tab-stops:list .5in'><![if !supportLists]>2)<span style='font:7.0pt "Times New Roman"'>&nbsp;&nbsp;&nbsp;
      | </span><![endif]>error vector <span style='font-family:Symbol;mso-ascii-font-family:
      | "Times New Roman";mso-hansi-font-family:"Times New Roman";mso-char-type:symbol;
      | mso-symbol-font-family:Symbol'><span style='mso-char-type:symbol;mso-symbol-font-family:
      | Symbol'>z</span></span> (<span style='font-family:Symbol;mso-ascii-font-family:
      | "Times New Roman";mso-hansi-font-family:"Times New Roman";mso-char-type:symbol;
      | mso-symbol-font-family:Symbol'><span style='mso-char-type:symbol;mso-symbol-font-family:
      | Symbol'>z</span></span>=ePb=(y-ys)Pb).</p>
      | 
      | <p class=MsoNormal style='margin-top:0in;margin-right:-1.8pt;margin-bottom:
      | 0in;margin-left:.5in;margin-bottom:.0001pt;text-indent:-.25in;mso-list:l2 level1 lfo2;
      | tab-stops:list .5in'><![if !supportLists]>3)<span style='font:7.0pt "Times New Roman"'>&nbsp;&nbsp;&nbsp;
      | </span><![endif]>Learning Enable LE, (Enables/Disables learning by
      | pre-multiplying e by 0 or 1)</p>
      | 
      | <p class=MsoNormal style='margin-right:-1.8pt'><![if !supportEmptyParas]>&nbsp;<![endif]><o:p></o:p></p>
      | 
      | <p class=MsoNormal style='margin-right:-1.8pt'>The <u>States</u> are all V and
      | W entries.</p>
      | 
      | <p class=MsoNormal style='margin-right:-1.8pt'><![if !supportEmptyParas]>&nbsp;<![endif]><o:p></o:p></p>
      | 
      | <p class=MsoNormal style='margin-right:-1.8pt;text-align:justify'>The <u>Outputs</u>
      | are:</p>
      | 
      | <p class=MsoNormal style='margin-top:0in;margin-right:-1.8pt;margin-bottom:
      | 0in;margin-left:.5in;margin-bottom:.0001pt;text-indent:-.25in;mso-list:l1 level1 lfo4;
      | tab-stops:list .5in'><![if !supportLists]>1)<span style='font:7.0pt "Times New Roman"'>&nbsp;&nbsp;&nbsp;
      | </span><![endif]>ys, neural network estimation , = v<sub>ad</sub> (adaptive
      | contribution) + v<sub>bar</sub> (robustifying contribution).</p>
      | 
      | <p class=MsoNormal style='margin-top:0in;margin-right:-1.8pt;margin-bottom:
      | 0in;margin-left:.5in;margin-bottom:.0001pt;text-indent:-.25in;mso-list:l1 level1 lfo4;
      | tab-stops:list .5in'><![if !supportLists]>2)<span style='font:7.0pt "Times New Roman"'>&nbsp;&nbsp;&nbsp;
      | </span><![endif]>X, Neural network state, composed by all W and V entries taken
      | columnwise.</p>
      | 
      | <p class=MsoNormal style='margin-right:-1.8pt'><![if !supportEmptyParas]>&nbsp;<![endif]><o:p></o:p></p>
      | 
      | <p class=MsoNormal style='margin-right:-1.8pt'>The <u>first</u> parameter must
      | be a vector containing:</p>
      | 
      | <p class=MsoNormal style='margin-top:0in;margin-right:-1.8pt;margin-bottom:
      | 0in;margin-left:.5in;margin-bottom:.0001pt;text-indent:-.25in;mso-list:l0 level1 lfo6;
      | tab-stops:list .5in'><![if !supportLists]>1)<span style='font:7.0pt "Times New Roman"'>&nbsp;&nbsp;&nbsp;
      | </span><![endif]>nno = number of network output = size of the error.</p>
      | 
      | <p class=MsoNormal style='margin-top:0in;margin-right:-1.8pt;margin-bottom:
      | 0in;margin-left:.5in;margin-bottom:.0001pt;text-indent:-.25in;mso-list:l0 level1 lfo6;
      | tab-stops:list .5in'><![if !supportLists]>2)<span style='font:7.0pt "Times New Roman"'>&nbsp;&nbsp;&nbsp;
      | </span><![endif]>nni = number of network inputs = plant states.</p>
      | 
      | <p class=MsoNormal style='margin-top:0in;margin-right:-1.8pt;margin-bottom:
      | 0in;margin-left:.5in;margin-bottom:.0001pt;text-indent:-.25in;mso-list:l0 level1 lfo6;
      | tab-stops:list .5in'><![if !supportLists]>3)<span style='font:7.0pt "Times New Roman"'>&nbsp;&nbsp;&nbsp;
      | </span><![endif]>nnh = number of hidden layer neurons.</p>
      | 
      | <p class=MsoNormal style='margin-right:-1.8pt'><![if !supportEmptyParas]>&nbsp;<![endif]><o:p></o:p></p>
      | 
      | <p class=MsoBodyText style='margin-right:-1.8pt'>The <u>second</u> parameter
      | must be a vector containing:</p>
      | 
      | <p class=MsoNormal style='margin-top:0in;margin-right:-1.8pt;margin-bottom:
      | 0in;margin-left:.5in;margin-bottom:.0001pt;text-indent:-.25in;mso-list:l3 level1 lfo8;
      | tab-stops:list .5in'><![if !supportLists]>1)<span style='font:7.0pt "Times New Roman"'>&nbsp;&nbsp;&nbsp;
      | </span><![endif]>G = learning rate of V (input layer).</p>
      | 
      | <p class=MsoNormal style='margin-top:0in;margin-right:-1.8pt;margin-bottom:
      | 0in;margin-left:.5in;margin-bottom:.0001pt;text-indent:-.25in;mso-list:l3 level1 lfo8;
      | tab-stops:list .5in'><![if !supportLists]>2)<span style='font:7.0pt "Times New Roman"'>&nbsp;&nbsp;&nbsp;
      | </span><![endif]>F = learning rate of W (output layer).</p>
      | 
      | <p class=MsoNormal style='margin-top:0in;margin-right:-1.8pt;margin-bottom:
      | 0in;margin-left:.5in;margin-bottom:.0001pt;text-indent:-.25in;mso-list:l3 level1 lfo8;
      | tab-stops:list .5in'><![if !supportLists]>3)<span style='font:7.0pt "Times New Roman"'>&nbsp;&nbsp;&nbsp;
      | </span><![endif]>lambda (e modification) = coefficient multiplying <span
      | style='font-family:Symbol;mso-ascii-font-family:"Times New Roman";mso-hansi-font-family:
      | "Times New Roman";mso-char-type:symbol;mso-symbol-font-family:Symbol'><span
      | style='mso-char-type:symbol;mso-symbol-font-family:Symbol'>z</span></span> in
      | the adaptation laws.</p>
      | 
      | <p class=MsoNormal style='margin-top:0in;margin-right:-1.8pt;margin-bottom:
      | 0in;margin-left:.5in;margin-bottom:.0001pt;text-indent:-.25in;mso-list:l3 level1 lfo8;
      | tab-stops:list .5in'><![if !supportLists]>4)<span style='font:7.0pt "Times New Roman"'>&nbsp;&nbsp;&nbsp;
      | </span><![endif]>act = sigmoid activation potential (supposed to be 1).</p>
      | 
      | <p class=MsoNormal style='margin-top:0in;margin-right:-1.8pt;margin-bottom:
      | 0in;margin-left:.5in;margin-bottom:.0001pt;text-indent:-.25in;mso-list:l3 level1 lfo8;
      | tab-stops:list .5in'><![if !supportLists]>5)<span style='font:7.0pt "Times New Roman"'>&nbsp;&nbsp;&nbsp;
      | </span><![endif]>bias = supposed to be 1, but could be 0 if the function to be
      | approximated has no constant component.</p>
      | 
      | <p class=MsoNormal style='margin-right:-1.8pt'><![if !supportEmptyParas]>&nbsp;<![endif]><o:p></o:p></p>
      | 
      | <p class=MsoNormal style='margin-right:-1.8pt'>The <u>third</u> parameter
      | contains limits for each element of the W and V matrices.</p>
      | 
      | <p class=MsoNormal style='margin-right:-1.8pt'>In other words, a limiting
      | mechanism is implemented within the code so that all the weights in W and V are always limited by the value entered in the mask.</p>
      | 
      | <p class=MsoNormal style='margin-right:-1.8pt'><![if !supportEmptyParas]>&nbsp;<![endif]><o:p></o:p></p>
      | 
      | <p class=MsoBodyText style='margin-right:-1.8pt'>The <u>fourth</u> parameter is
      | related to the robustifying term and must be a vector containing:</p>
      | 
      | <p class=MsoNormal style='margin-top:0in;margin-right:-1.8pt;margin-bottom:
      | 0in;margin-left:.5in;margin-bottom:.0001pt;text-indent:-.25in;mso-list:l4 level1 lfo10;
      | tab-stops:list .5in'><![if !supportLists]>1)<span style='font:7.0pt "Times New Roman"'>&nbsp;&nbsp;&nbsp;
      | </span><![endif]>K<sub>v</sub> = multiplies first term of v<sub>bar</sub>.</p>
      | 
      | <p class=MsoNormal style='margin-top:0in;margin-right:-1.8pt;margin-bottom:
      | 0in;margin-left:.5in;margin-bottom:.0001pt;text-indent:-.25in;mso-list:l4 level1 lfo10;
      | tab-stops:list .5in'><![if !supportLists]>2)<span style='font:7.0pt "Times New Roman"'>&nbsp;&nbsp;&nbsp;
      | </span><![endif]>Z<sub>bar</sub> = maximum expected <span style='font-family:
      | Symbol;mso-ascii-font-family:"Times New Roman";mso-hansi-font-family:"Times New Roman";
      | mso-char-type:symbol;mso-symbol-font-family:Symbol'><span style='mso-char-type:
      | symbol;mso-symbol-font-family:Symbol'>ï</span></span>Z<span style='font-family:
      | Symbol;mso-ascii-font-family:"Times New Roman";mso-hansi-font-family:"Times New Roman";
      | mso-char-type:symbol;mso-symbol-font-family:Symbol'><span style='mso-char-type:
      | symbol;mso-symbol-font-family:Symbol'>ï</span></span><sub>F</sub> value (see v<sub>bar</sub>).</p>
      | 
      | <p class=MsoNormal style='margin-top:0in;margin-right:-1.8pt;margin-bottom:
      | 0in;margin-left:.5in;margin-bottom:.0001pt;text-indent:-.25in;mso-list:l4 level1 lfo10;
      | tab-stops:list .5in'><![if !supportLists]>3)<span style='font:7.0pt "Times New Roman"'>&nbsp;&nbsp;&nbsp;
      | </span><![endif]>K<sub>z</sub> = multiplies second term of v<sub>bar</sub>.</p>
      | 
      | <p class=MsoNormal style='margin-right:-1.8pt'><![if !supportEmptyParas]>&nbsp;<![endif]><o:p></o:p></p>
      | 
      | <p class=MsoNormal style='margin-right:-1.8pt'>The <u>fifth</u> and <u>sixth</u>
      | parameter contain initial conditions for the Matrices W and W.</p>
      | 
      | <p class=MsoNormal style='margin-right:-1.8pt'><![if !supportEmptyParas]>&nbsp;<![endif]><o:p></o:p></p>
      | 
      | <p class=MsoNormal style='margin-right:-1.8pt'>Finally, the last parameter is
      | the sampling time of the discrete-time integrator.</p>
      | 
      | <p class=MsoNormal style='margin-right:-1.8pt'><![if !supportEmptyParas]>&nbsp;<![endif]><o:p></o:p></p>
      | 
      | <p class=MsoNormal style='margin-right:-1.8pt'>G.Campa, January 2007, West
      | Virginia University</p>
      | 
      | </div>
      | 
      | </body>
      | 
      | </html>
  Pid Demo F4 : Subsystem
      settings: OpenFcn=anndemo
      mask Display: disp('ANN\nDemo')
